simulink model "Robot_control"  (Simulink 9.0)
settings: Solver=ode45  StartTime=0.0  StopTime=100  RelTol=1e-3
libraries: mblibv1 x4, simulink x2, vrlib x1
settings Model: Creator=zigg  LastModifiedBy=alinvoicu26
settings DataIOCC: SaveFormat=StructureWithTime
settings DebuggingCC: UnderspecifiedInitializationDetection=Simplified  MergeDetectMultiDrivingBlocksExec=error  FcnCallInpInsideContextMsg=warning  SFUnexpectedBacktrackingDiag=error  SFNoUnconditionalDefaultTransitionDiag=error
settings HardwareCC: ProdBitPerPointer=64  ProdLargestAtomicFloat=Float  ProdIntDivRoundTo=Zero  ProdEndianess=LittleEndian  ProdHWDeviceType=Specified
settings ModelReferenceCC: PropagateSignalLabelsOutOfModel=on
settings GRTTargetCC: TargetLangStandard=C99 (ISO)
settings ConfigComp: CovMetricSettings=dwe  CovHtmlReporting=off  CovSaveCumulativeToWorkspaceVar=off  CovSaveSingleToWorkspaceVar=off  CovExternalEMLEnable=on

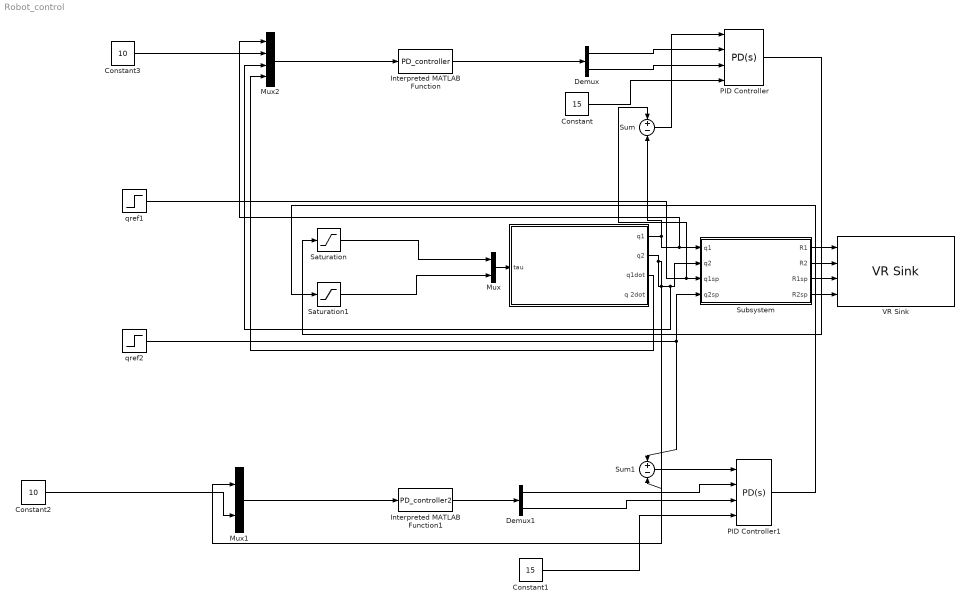
== system Robot_control ==
  "  " : Subsystem
  Constant : Constant  Value=15
  Constant1 : Constant  Value=15
  Constant2 : Constant  Value=10
  Constant3 : Constant  Value=10
  Demux : Demux  Outputs=2
  Demux1 : Demux  Outputs=2
  Interpreted MATLAB Function : MATLABFcn  MATLABFcn=PD_controller  OutputDimensions=2
  Interpreted MATLAB Function1 : MATLABFcn  MATLABFcn=PD_controller2  OutputDimensions=2
  Mux : Mux  Inputs=2
  Mux1 : Mux  Inputs=2
  Mux2 : Mux
  PID Controller : simulink/Continuous/PID Controller  Controller=PD  TimeDomain=Continuous-time  SampleTime=-1  IntegratorMethod=Forward Euler  FilterMethod=Forward Euler  Form=Parallel  UseFilter=on  ControllerParametersSource=external  P=1  I=1  D=0  N=100  InitialConditionSource=internal  InitialConditionForIntegrator=0  InitialConditionForFilter=0  ExternalReset=none  LimitOutput=off  UpperSaturationLimit=inf  LowerSaturationLimit=-inf  LinearizeAsGain=on  AntiWindupMode=none  Kb=1  TrackingMode=off  Kt=1  PParamMin=[]  PParamMax=[]  IParamMin=[]  IParamMax=[]  DParamMin=[]  DParamMax=[]  NParamMin=[]  NParamMax=[]  KbParamMin=[]  KbParamMax=[]  KtParamMin=[]  KtParamMax=[]  POutMin=[]  POutMax=[]  IOutMin=[]  IOutMax=[]  DOutMin=[]  DOutMax=[]  NOutMin=[]  NOutMax=[]  KbOutMin=[]  KbOutMax=[]  KtOutMin=[]  KtOutMax=[]  IntegratorOutMin=[]  IntegratorOutMax=[]  FilterOutMin=[]  FilterOutMax=[]  SumOutMin=[]  SumOutMax=[]  SumI1OutMin=[]  SumI1OutMax=[]  SumI2OutMin=[]  SumI2OutMax=[]  SumI3OutMin=[]  SumI3OutMax=[]  SumDOutMin=[]  SumDOutMax=[]  SaturationOutMin=[]  SaturationOutMax=[]  IntegratorContinuousStateAttributes=''  IntegratorStateMustResolveToSignalObject=off  IntegratorRTWStateStorageClass=Auto  FilterContinuousStateAttributes=''  FilterStateMustResolveToSignalObject=off  FilterRTWStateStorageClass=Auto  DifferentiatorICPrevScaledInput=0  DifferentiatorOutMin=[]  DifferentiatorOutMax=[]  InitialConditionSetting=State (most efficient)  FilterDiffOutCoefMin=[]  FilterDiffOutCoefMax=[]  SumDenOutMin=[]  SumDenOutMax=[]  SumNumOutMin=[]  SumNumOutMax=[]  ReciprocalOutMin=[]  ReciprocalOutMax=[]  DivideOutMin=[]  DivideOutMax=[]  TunerSelectOption=Transfer Function Based (PID Tuner App)
  PID Controller1 : simulink/Continuous/PID Controller  Controller=PD  TimeDomain=Continuous-time  SampleTime=-1  IntegratorMethod=Forward Euler  FilterMethod=Forward Euler  Form=Parallel  UseFilter=on  ControllerParametersSource=external  P=1  I=1  D=0  N=100  InitialConditionSource=internal  InitialConditionForIntegrator=0  InitialConditionForFilter=0  ExternalReset=none  LimitOutput=off  UpperSaturationLimit=inf  LowerSaturationLimit=-inf  LinearizeAsGain=on  AntiWindupMode=none  Kb=1  TrackingMode=off  Kt=1  PParamMin=[]  PParamMax=[]  IParamMin=[]  IParamMax=[]  DParamMin=[]  DParamMax=[]  NParamMin=[]  NParamMax=[]  KbParamMin=[]  KbParamMax=[]  KtParamMin=[]  KtParamMax=[]  POutMin=[]  POutMax=[]  IOutMin=[]  IOutMax=[]  DOutMin=[]  DOutMax=[]  NOutMin=[]  NOutMax=[]  KbOutMin=[]  KbOutMax=[]  KtOutMin=[]  KtOutMax=[]  IntegratorOutMin=[]  IntegratorOutMax=[]  FilterOutMin=[]  FilterOutMax=[]  SumOutMin=[]  SumOutMax=[]  SumI1OutMin=[]  SumI1OutMax=[]  SumI2OutMin=[]  SumI2OutMax=[]  SumI3OutMin=[]  SumI3OutMax=[]  SumDOutMin=[]  SumDOutMax=[]  SaturationOutMin=[]  SaturationOutMax=[]  IntegratorContinuousStateAttributes=''  IntegratorStateMustResolveToSignalObject=off  IntegratorRTWStateStorageClass=Auto  FilterContinuousStateAttributes=''  FilterStateMustResolveToSignalObject=off  FilterRTWStateStorageClass=Auto  DifferentiatorICPrevScaledInput=0  DifferentiatorOutMin=[]  DifferentiatorOutMax=[]  InitialConditionSetting=State (most efficient)  FilterDiffOutCoefMin=[]  FilterDiffOutCoefMax=[]  SumDenOutMin=[]  SumDenOutMax=[]  SumNumOutMin=[]  SumNumOutMax=[]  ReciprocalOutMin=[]  ReciprocalOutMax=[]  DivideOutMin=[]  DivideOutMax=[]  TunerSelectOption=Transfer Function Based (PID Tuner App)
  Saturation : Saturate  UpperLimit=1.18  LowerLimit=-1.18
  Saturation1 : Saturate  UpperLimit=1.18  LowerLimit=-1.18
  Subsystem : Subsystem
  Sum : Sum  Inputs=+-
  Sum1 : Sum  Inputs=+-
  VR Sink : vrlib/VR Sink  InstantiateOnLoad=on  SampleTime=0.1  ViewEnable=on  RemoteChange=off  RemoteView=off  FieldsWritten=Joint1.rotation.4.1.1.double#Joint2.rotation.4.1.1.double#Joint1_SP.rotation.4.1.1.double#Joint2_SP.rotation.4.1.1.double  WorldFileName=my_robot.wrl  AutoView=off  VideoDimensions=[]  AllowVariableSize=off
      settings: SourceProductBaseCode=VR
  qref1 : Step  SampleTime=0
  qref2 : Step  SampleTime=0
  wires:
  Subsystem/1(R1) -> VR Sink/1
  Subsystem/2(R2) -> VR Sink/2
  Subsystem/3(R1sp) -> VR Sink/3
  Subsystem/4(R2sp) -> VR Sink/4
  "  "/1(q1) -> Mux2/1, Subsystem/1(q1), Sum/2
  qref2/1 -> Subsystem/4(q2sp), Sum1/1
  qref1/1 -> Sum/1, Subsystem/3(q1sp)
  Mux/1 -> "  "/1(tau)
  Saturation1/1 -> Mux/2
  Saturation/1 -> Mux/1
  PID Controller/1 -> Saturation/1
  PID Controller1/1 -> Saturation1/1
  Sum1/1 -> PID Controller1/1
  "  "/2(q2) -> Mux1/1, Sum1/2, Mux2/3, Subsystem/2(q2)
  Interpreted MATLAB Function1/1 -> Demux1/1
  Demux1/1 -> PID Controller1/2
  Demux1/2 -> PID Controller1/3
  Constant1/1 -> PID Controller1/4
  Constant2/1 -> Mux1/2
  Mux1/1 -> Interpreted MATLAB Function1/1
  Demux/1 -> PID Controller/2
  Demux/2 -> PID Controller/3
  Sum/1 -> PID Controller/1
  Constant/1 -> PID Controller/4
  Interpreted MATLAB Function/1 -> Demux/1
  Mux2/1 -> Interpreted MATLAB Function/1
  Constant3/1 -> Mux2/2
  "  "/3(q1dot) -> Mux2/4

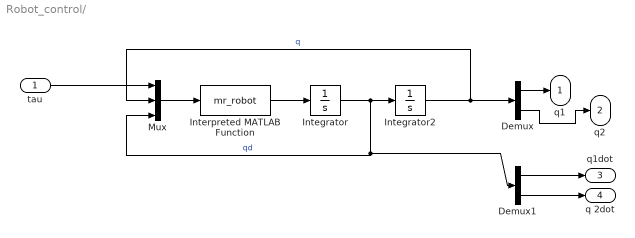
== system Robot_control/   ==
  tau : Inport
  Demux : Demux  Outputs=2
  Demux1 : Demux  Outputs=2
  Integrator : Integrator
  Integrator2 : Integrator  InitialCondition=pi/2*0
  Interpreted MATLAB Function : MATLABFcn  MATLABFcn=mr_robot  OutputDimensions=2
  Mux : Mux  Inputs=3
  q1 : Outport
  q2 : Outport  Port=2
  q1dot : Outport  Port=3
  "q 2dot " : Outport  Port=4
  wires:
  Interpreted MATLAB Function/1 -> Integrator/1
  Integrator2/1 -> Demux/1, Mux/2  "q"
  Integrator/1 -> Demux1/1, Mux/3, Integrator2/1  "qd"
  tau/1 -> Mux/1
  Mux/1 -> Interpreted MATLAB Function/1
  Demux/1 -> q1/1
  Demux/2 -> q2/1
  Demux1/1 -> q1dot/1
  Demux1/2 -> "q 2dot "/1

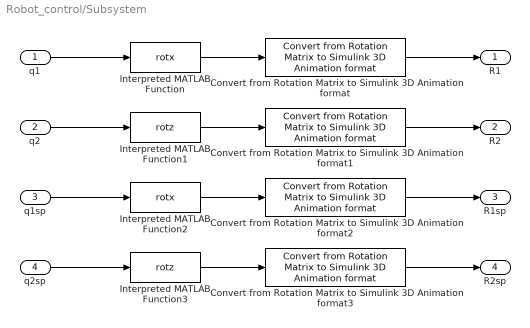
== system Robot_control/Subsystem ==
  q1 : Inport
  q2 : Inport  Port=2
  q1sp : Inport  Port=3
  q2sp : Inport  Port=4
  Convert from Rotation Matrix to Simulink 3D Animation format{,1..3} (4 alike) : mblibv1/Utilities/Convert from Rotation Matrix to Simulink 3D Animation format
      settings: SourceProductName=Simscape Multibody  SourceProductBaseCode=MS
  Interpreted MATLAB Function : MATLABFcn  MATLABFcn=rotx
  Interpreted MATLAB Function1 : MATLABFcn  MATLABFcn=rotz
  Interpreted MATLAB Function2 : MATLABFcn  MATLABFcn=rotx
  Interpreted MATLAB Function3 : MATLABFcn  MATLABFcn=rotz
  R1 : Outport
  R2 : Outport  Port=2
  R1sp : Outport  Port=3
  R2sp : Outport  Port=4
  wires:
  Convert from Rotation Matrix to Simulink 3D Animation format/1 -> R1/1
  Interpreted MATLAB Function/1 -> Convert from Rotation Matrix to Simulink 3D Animation format/1
  Interpreted MATLAB Function1/1 -> Convert from Rotation Matrix to Simulink 3D Animation format1/1
  Interpreted MATLAB Function2/1 -> Convert from Rotation Matrix to Simulink 3D Animation format2/1
  Interpreted MATLAB Function3/1 -> Convert from Rotation Matrix to Simulink 3D Animation format3/1
  q1/1 -> Interpreted MATLAB Function/1
  q2/1 -> Interpreted MATLAB Function1/1
  q1sp/1 -> Interpreted MATLAB Function2/1
  q2sp/1 -> Interpreted MATLAB Function3/1
  Convert from Rotation Matrix to Simulink 3D Animation format1/1 -> R2/1
  Convert from Rotation Matrix to Simulink 3D Animation format2/1 -> R1sp/1
  Convert from Rotation Matrix to Simulink 3D Animation format3/1 -> R2sp/1
